simulink model "robocar_ss"  (R2024b)
settings: Solver=FixedStepAuto  StartTime=0  StopTime=5  FixedStep=0.001  RelTol=1e-3
libraries: slpidlib x4
settings Model: Creator=saucesaft  LastModifiedBy=saucesaft
settings HardwareCC: ProdBitPerLong=64  ProdHWDeviceType=Apple->ARM64

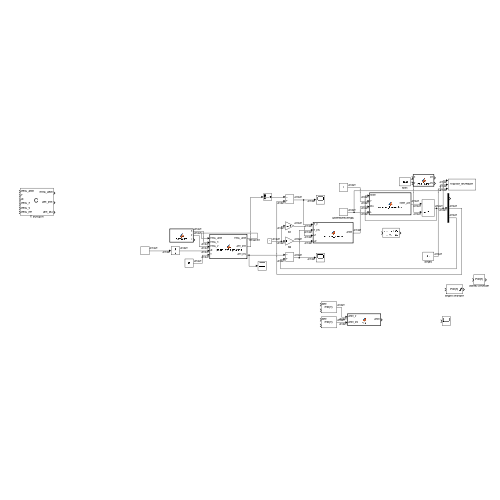
[thumbnail: Simulink's stored preview of the top-level diagram]
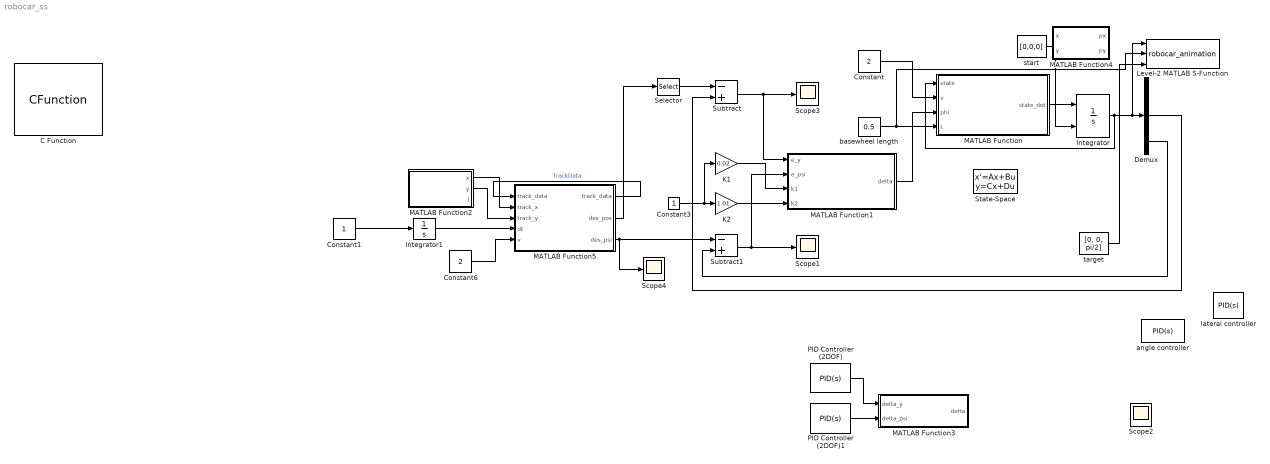
== system robocar_ss ==
  C Function : CFunction  OutputCode=|  InitializeConditionsCode=init = true;  CodegenOutputCode=|  CodegenInitializeConditionsCode=init = true;  SampleTime=0.01  CustomCodeSettingLocation=ModelConfigurationParameters
      OutputCode=|
      | #define MAX(x, y) (((x) > (y)) ? (x) : (y))
      | #define MIN(x, y) (((x) < (y)) ? (x) : (y))
      | 
      | if (init) {
      |     track_data.index = 1;
      |     track_data.t_marker = 0;
      | 
      |     track_data.A[0] = track_x[0];
      |     track_data.A[1] = track_y[0];
      | 
      |     track_data.B[0] = track_x[1];
      |     track_data.B[1] = track_y[1];
      |     
      |     init = false;
      | } 
      | 
      | double mag_vector[2];
      | mag_vector[0] = track_data.des_pos[0] - track_data.A[0];
      | mag_vector[1] = track_data.des_pos[1] - track_data.A[1];
      | 
      | double mag = sqrt( pow(mag_vector[0], 2) + pow(mag_vector[1], 2) );
      | 
      | if (mag >= track_data.base_norm) {
      |     track_data.index = MIN(track_data.index+1, track_len-1);
      |     
      |     mag_vector[0] = track_data.des_pos[0] - track_data.B[0];
      |     mag_vector[1] = track_data.des_pos[1] - track_data.B[1];
      |     track_data.t_marker = dt - (sqrt( pow(mag_vector[0], 2) + pow(mag_vector[1], 2) )/v);
      |     
      |     track_data.A[0] = track_x[track_data.index];
      |     track_data.A[1] = track_y[track_data.index];
      |     
      |     track_data.B[0] = track_x[track_data.index + 1];
      |     track_data.B[1] = track_y[track_data.index + 1];
      |     
      |     mag_vector[0] = track_data.B[0] - track_data.A[0];
      |     mag_vector[1] = track_data.B[1] - track_data.A[1];
      |     track_data.base_norm = sqrt( pow(mag_vector[0], 2) + pow(mag_vector[1], 2) );
      | }
      | 
      | mag_vector[0] = track_data.B[0] - track_data.A[0];
      | mag_vector[1] = track_data.B[1] - track_data.A[1];
      | mag = sqrt( pow(mag_vector[0], 2) + pow(mag_vector[1], 2) );
      | 
      | track_data.des_pos[0] = track_data.A[0] + v*(dt - track_data.t_marker) * (track_data.B[0]-track_data.A[0]) / mag;
      | track_data.des_pos[1] = track_data.A[1] + v*(dt - track_data.t_marker) * (track_data.B[1]-track_data.A[1]) / mag;
      | 
      | des_pos[0] = track_data.des_pos[0];
      | des_pos[1] = track_data.des_pos[1];
      | des_phi = atan2( track_data.B[1] - track_data.A[1], track_data.B[0] - track_data.A[0] );
      CodegenOutputCode=|
      | #define MAX(x, y) (((x) > (y)) ? (x) : (y))
      | #define MIN(x, y) (((x) < (y)) ? (x) : (y))
      | 
      | if (init) {
      |     track_data.index = 1;
      |     track_data.t_marker = 0;
      | 
      |     track_data.A[0] = track_x[0];
      |     track_data.A[1] = track_y[0];
      | 
      |     track_data.B[0] = track_x[1];
      |     track_data.B[1] = track_y[1];
      |     
      |     init = false;
      | } 
      | 
      | double mag_vector[2];
      | mag_vector[0] = track_data.des_pos[0] - track_data.A[0];
      | mag_vector[1] = track_data.des_pos[1] - track_data.A[1];
      | 
      | double mag = sqrt( pow(mag_vector[0], 2) + pow(mag_vector[1], 2) );
      | 
      | if (mag >= track_data.base_norm) {
      |     track_data.index = MIN(track_data.index+1, track_len-1);
      |     
      |     mag_vector[0] = track_data.des_pos[0] - track_data.B[0];
      |     mag_vector[1] = track_data.des_pos[1] - track_data.B[1];
      |     track_data.t_marker = dt - (sqrt( pow(mag_vector[0], 2) + pow(mag_vector[1], 2) )/v);
      |     
      |     track_data.A[0] = track_x[track_data.index];
      |     track_data.A[1] = track_y[track_data.index];
      |     
      |     track_data.B[0] = track_x[track_data.index + 1];
      |     track_data.B[1] = track_y[track_data.index + 1];
      |     
      |     mag_vector[0] = track_data.B[0] - track_data.A[0];
      |     mag_vector[1] = track_data.B[1] - track_data.A[1];
      |     track_data.base_norm = sqrt( pow(mag_vector[0], 2) + pow(mag_vector[1], 2) );
      | }
      | 
      | mag_vector[0] = track_data.B[0] - track_data.A[0];
      | mag_vector[1] = track_data.B[1] - track_data.A[1];
      | mag = sqrt( pow(mag_vector[0], 2) + pow(mag_vector[1], 2) );
      | 
      | track_data.des_pos[0] = track_data.A[0] + v*(dt - track_data.t_marker) * (track_data.B[0]-track_data.A[0]) / mag;
      | track_data.des_pos[1] = track_data.A[1] + v*(dt - track_data.t_marker) * (track_data.B[1]-track_data.A[1]) / mag;
      | 
      | des_pos[0] = track_data.des_pos[0];
      | des_pos[1] = track_data.des_pos[1];
      | des_phi = atan2( track_data.B[1] - track_data.A[1], track_data.B[0] - track_data.A[0] );
  Constant : Constant  Value=2
  Constant1 : Constant
  Constant3 : Constant
  Constant6 : Constant  Value=2
  Demux : Demux  Outputs=3
  Integrator : Integrator  InitialConditionSource=external  InitialCondition=[5,10,pi]
  Integrator1 : Integrator
  K1 : Gain  Gain=0.02
  K2 : Gain  Gain=1.01
  Level-2 MATLAB S-Function : M-S-Function  FunctionName=robocar_animation
  MATLAB Function : MATLAB Function  TreatAsAtomicUnit=on
  MATLAB Function1 : MATLAB Function  TreatAsAtomicUnit=on
  MATLAB Function2 : MATLAB Function  TreatAsAtomicUnit=on
  MATLAB Function3 : MATLAB Function  TreatAsAtomicUnit=on
  MATLAB Function4 : MATLAB Function  TreatAsAtomicUnit=on
  MATLAB Function5 : MATLAB Function  TreatAsAtomicUnit=on
  PID Controller (2DOF) : slpidlib/PID Controller (2DOF)  Controller=PID  Form=Parallel  TimeDomain=Continuous-time  UseExternalTs=off  SampleTime=-1  IntegratorMethod=Forward Euler  FilterMethod=Forward Euler  ControllerParametersSource=internal  P=1  I=1  UseKiTs=off  D=0  UseExternalDerivativeSource=off  N=100  UseFilter=on  b=1  c=1  TunerSelectOption=Transfer Function Based (PID Tuner App)  InitialConditionSource=internal  InitialConditionForIntegrator=0  InitialConditionForFilter=0  DifferentiatorICPrevScaledInput=0  ExternalReset=none  TrackingMode=off  Kt=1  LimitOutput=off  SatLimitsSource=internal  UpperSaturationLimit=inf  LowerSaturationLimit=-inf  LinearizeAsGain=on  AntiWindupMode=none  Kb=1  LimitIntegrator=off  UpperIntegratorSaturationLimit=inf  LowerIntegratorSaturationLimit=-inf  POutMin=[]  POutMax=[]  IOutMin=[]  IOutMax=[]  DOutMin=[]  DOutMax=[]  NOutMin=[]  NOutMax=[]  bOutMin=[]  bOutMax=[]  cOutMin=[]  cOutMax=[]  SumOutMin=[]  SumOutMax=[]  SaturationOutMin=[]  SaturationOutMax=[]  PParamMin=[]  PParamMax=[]  IParamMin=[]  IParamMax=[]  DParamMin=[]  DParamMax=[]  NParamMin=[]  NParamMax=[]  bParamMin=[]  bParamMax=[]  cParamMin=[]  cParamMax=[]  KbParamMin=[]  KbParamMax=[]  KtParamMin=[]  KtParamMax=[]  KbOutMin=[]  KbOutMax=[]  KtOutMin=[]  KtOutMax=[]  IntegratorOutMin=[]  IntegratorOutMax=[]  FilterOutMin=[]  FilterOutMax=[]  SumI1OutMin=[]  SumI1OutMax=[]  SumI2OutMin=[]  SumI2OutMax=[]  SumI3OutMin=[]  SumI3OutMax=[]  SumI4OutMin=[]  SumI4OutMax=[]  SumDOutMin=[]  SumDOutMax=[]  Sum1OutMin=[]  Sum1OutMax=[]  Sum2OutMin=[]  Sum2OutMax=[]  Sum3OutMin=[]  Sum3OutMax=[]  DifferentiatorOutMin=[]  DifferentiatorOutMax=[]  FilterDiffOutCoefMin=[]  FilterDiffOutCoefMax=[]  ReciprocalOutMin=[]  ReciprocalOutMax=[]  SumDenOutMin=[]  SumDenOutMax=[]  SumNumOutMin=[]  SumNumOutMax=[]  DivideOutMin=[]  DivideOutMax=[]  UdiffTsProdOutMin=[]  UdiffTsProdOutMax=[]  NTsProdOutMin=[]  NTsProdOutMax=[]  UintegralTsProdOutMin=[]  UintegralTsProdOutMax=[]  UngainTsProdOutMin=[]  UngainTsProdOutMax=[]  ClampingZeroOutDataTypeStr=Inherit: Inherit via back propagation  ClampingZeroOutMin=[]  ClampingZeroOutMax=[]  FilterDenConstantOutDataTypeStr=Inherit: Inherit via back propagation  FilterDenConstantOutMin=[]  FilterDenConstantOutMax=[]  PCopyOutDataTypeStr=Inherit: Inherit via back propagation  PCopyOutMin=[]  PCopyOutMax=[]  NCopyOutDataTypeStr=Inherit: Inherit via back propagation  NCopyOutMin=[]  NCopyOutMax=[]  IntegratorContinuousStateAttributes=''  IntegratorStateMustResolveToSignalObject=off  IntegratorRTWStateStorageClass=Auto  FilterContinuousStateAttributes=''  FilterStateMustResolveToSignalObject=off  FilterRTWStateStorageClass=Auto  ParallelPVariant=InternalParameters  IdealPVariant=Disabled  IVariant=InternalParameters  DVariant=InternalParameters  bVariant=InternalParameters  cVariant=InternalParameters  IntegratorVariant=Continuous  SatVariant=Disabled  AWVariant=Passthrough  PCopyVariant=Disabled  TRVariant=Disabled  FdbkBlocksVariant=Forward  IdealPFdbkVariant=Disabled  SatFdbkVariant=Disabled  DerivativeFilterVariant=ContFilter  NVariant=InternalParameters  NCopyVariant=Disabled  FilterICVariant=InternalICsFilter  IntegratorICVariant=InternalICs  ExternalResetVariant=Disabled  TRSumVariant=Passthrough  SumFdbkVariant=Disabled  SumVariant=Sum_PID  TsampFilterVariant=InternalTs  TsampNgainVariant=Passthrough  TsampIntegralVariant=Disabled_SignalSpec  ExternalSaturationOutDataTypeStr=Inherit: Same as second input  DerivativeSourceVariant=ErrorSignal  PreIntVariant=InternalPreInt
  PID Controller (2DOF)1 : slpidlib/PID Controller (2DOF)  Controller=PID  Form=Parallel  TimeDomain=Continuous-time  UseExternalTs=off  SampleTime=-1  IntegratorMethod=Forward Euler  FilterMethod=Forward Euler  ControllerParametersSource=internal  P=1  I=1  UseKiTs=off  D=0  UseExternalDerivativeSource=off  N=100  UseFilter=on  b=1  c=1  TunerSelectOption=Transfer Function Based (PID Tuner App)  InitialConditionSource=internal  InitialConditionForIntegrator=0  InitialConditionForFilter=0  DifferentiatorICPrevScaledInput=0  ExternalReset=none  TrackingMode=off  Kt=1  LimitOutput=off  SatLimitsSource=internal  UpperSaturationLimit=inf  LowerSaturationLimit=-inf  LinearizeAsGain=on  AntiWindupMode=none  Kb=1  LimitIntegrator=off  UpperIntegratorSaturationLimit=inf  LowerIntegratorSaturationLimit=-inf  POutMin=[]  POutMax=[]  IOutMin=[]  IOutMax=[]  DOutMin=[]  DOutMax=[]  NOutMin=[]  NOutMax=[]  bOutMin=[]  bOutMax=[]  cOutMin=[]  cOutMax=[]  SumOutMin=[]  SumOutMax=[]  SaturationOutMin=[]  SaturationOutMax=[]  PParamMin=[]  PParamMax=[]  IParamMin=[]  IParamMax=[]  DParamMin=[]  DParamMax=[]  NParamMin=[]  NParamMax=[]  bParamMin=[]  bParamMax=[]  cParamMin=[]  cParamMax=[]  KbParamMin=[]  KbParamMax=[]  KtParamMin=[]  KtParamMax=[]  KbOutMin=[]  KbOutMax=[]  KtOutMin=[]  KtOutMax=[]  IntegratorOutMin=[]  IntegratorOutMax=[]  FilterOutMin=[]  FilterOutMax=[]  SumI1OutMin=[]  SumI1OutMax=[]  SumI2OutMin=[]  SumI2OutMax=[]  SumI3OutMin=[]  SumI3OutMax=[]  SumI4OutMin=[]  SumI4OutMax=[]  SumDOutMin=[]  SumDOutMax=[]  Sum1OutMin=[]  Sum1OutMax=[]  Sum2OutMin=[]  Sum2OutMax=[]  Sum3OutMin=[]  Sum3OutMax=[]  DifferentiatorOutMin=[]  DifferentiatorOutMax=[]  FilterDiffOutCoefMin=[]  FilterDiffOutCoefMax=[]  ReciprocalOutMin=[]  ReciprocalOutMax=[]  SumDenOutMin=[]  SumDenOutMax=[]  SumNumOutMin=[]  SumNumOutMax=[]  DivideOutMin=[]  DivideOutMax=[]  UdiffTsProdOutMin=[]  UdiffTsProdOutMax=[]  NTsProdOutMin=[]  NTsProdOutMax=[]  UintegralTsProdOutMin=[]  UintegralTsProdOutMax=[]  UngainTsProdOutMin=[]  UngainTsProdOutMax=[]  ClampingZeroOutDataTypeStr=Inherit: Inherit via back propagation  ClampingZeroOutMin=[]  ClampingZeroOutMax=[]  FilterDenConstantOutDataTypeStr=Inherit: Inherit via back propagation  FilterDenConstantOutMin=[]  FilterDenConstantOutMax=[]  PCopyOutDataTypeStr=Inherit: Inherit via back propagation  PCopyOutMin=[]  PCopyOutMax=[]  NCopyOutDataTypeStr=Inherit: Inherit via back propagation  NCopyOutMin=[]  NCopyOutMax=[]  IntegratorContinuousStateAttributes=''  IntegratorStateMustResolveToSignalObject=off  IntegratorRTWStateStorageClass=Auto  FilterContinuousStateAttributes=''  FilterStateMustResolveToSignalObject=off  FilterRTWStateStorageClass=Auto  ParallelPVariant=InternalParameters  IdealPVariant=Disabled  IVariant=InternalParameters  DVariant=InternalParameters  bVariant=InternalParameters  cVariant=InternalParameters  IntegratorVariant=Continuous  SatVariant=Disabled  AWVariant=Passthrough  PCopyVariant=Disabled  TRVariant=Disabled  FdbkBlocksVariant=Forward  IdealPFdbkVariant=Disabled  SatFdbkVariant=Disabled  DerivativeFilterVariant=ContFilter  NVariant=InternalParameters  NCopyVariant=Disabled  FilterICVariant=InternalICsFilter  IntegratorICVariant=InternalICs  ExternalResetVariant=Disabled  TRSumVariant=Passthrough  SumFdbkVariant=Disabled  SumVariant=Sum_PID  TsampFilterVariant=InternalTs  TsampNgainVariant=Passthrough  TsampIntegralVariant=Disabled_SignalSpec  ExternalSaturationOutDataTypeStr=Inherit: Same as second input  DerivativeSourceVariant=ErrorSignal  PreIntVariant=InternalPreInt
  Scope{1..4} (4 alike) : Scope
  Selector : Selector  InputPortWidth=2  IndexOptions=Index vector (dialog)  Indices=2  OutputSizes=1
  State-Space : StateSpace  A=[0 10; 0 0]  B=[0; 10/1]  C=[1 0; 0 1]  D=[0; 0]  InitialCondition=0
  Subtract : Sum  Inputs=-+
  Subtract1 : Sum  Inputs=-+
  angle controller : slpidlib/PID Controller  Controller=PID  Form=Parallel  TimeDomain=Continuous-time  UseExternalTs=off  SampleTime=-1  IntegratorMethod=Forward Euler  FilterMethod=Forward Euler  ControllerParametersSource=internal  P=9.67739961508882  I=0.240279452636177  UseKiTs=off  D=100.4861253643554  UseExternalDerivativeSource=off  N=100  UseFilter=on  TunerSelectOption=Transfer Function Based (PID Tuner App)  InitialConditionSource=internal  InitialConditionForIntegrator=0  InitialConditionForFilter=0  DifferentiatorICPrevScaledInput=0  ExternalReset=none  TrackingMode=off  Kt=1  LimitOutput=on  SatLimitsSource=internal  UpperSaturationLimit=inf  LowerSaturationLimit=-inf  LinearizeAsGain=on  AntiWindupMode=back-calculation  Kb=1  LimitIntegrator=off  UpperIntegratorSaturationLimit=inf  LowerIntegratorSaturationLimit=-inf  POutMin=[]  POutMax=[]  IOutMin=[]  IOutMax=[]  DOutMin=[]  DOutMax=[]  NOutMin=[]  NOutMax=[]  SumOutMin=[]  SumOutMax=[]  SaturationOutMin=[]  SaturationOutMax=[]  PParamMin=[]  PParamMax=[]  IParamMin=[]  IParamMax=[]  DParamMin=[]  DParamMax=[]  NParamMin=[]  NParamMax=[]  KbParamMin=[]  KbParamMax=[]  KtParamMin=[]  KtParamMax=[]  KbOutMin=[]  KbOutMax=[]  KtOutMin=[]  KtOutMax=[]  IntegratorOutMin=[]  IntegratorOutMax=[]  FilterOutMin=[]  FilterOutMax=[]  SumI1OutMin=[]  SumI1OutMax=[]  SumI2OutMin=[]  SumI2OutMax=[]  SumI3OutMin=[]  SumI3OutMax=[]  SumI4OutMin=[]  SumI4OutMax=[]  SumDOutMin=[]  SumDOutMax=[]  DifferentiatorOutMin=[]  DifferentiatorOutMax=[]  FilterDiffOutCoefMin=[]  FilterDiffOutCoefMax=[]  ReciprocalOutMin=[]  ReciprocalOutMax=[]  SumDenOutMin=[]  SumDenOutMax=[]  SumNumOutMin=[]  SumNumOutMax=[]  DivideOutMin=[]  DivideOutMax=[]  UdiffTsProdOutMin=[]  UdiffTsProdOutMax=[]  NTsProdOutMin=[]  NTsProdOutMax=[]  UintegralTsProdOutMin=[]  UintegralTsProdOutMax=[]  UngainTsProdOutMin=[]  UngainTsProdOutMax=[]  ClampingZeroOutDataTypeStr=Inherit: Inherit via back propagation  ClampingZeroOutMin=[]  ClampingZeroOutMax=[]  FilterDenConstantOutDataTypeStr=Inherit: Inherit via back propagation  FilterDenConstantOutMin=[]  FilterDenConstantOutMax=[]  PCopyOutDataTypeStr=Inherit: Inherit via back propagation  PCopyOutMin=[]  PCopyOutMax=[]  NCopyOutDataTypeStr=Inherit: Inherit via back propagation  NCopyOutMin=[]  NCopyOutMax=[]  IntegratorContinuousStateAttributes=''  IntegratorStateMustResolveToSignalObject=off  IntegratorRTWStateStorageClass=Auto  FilterContinuousStateAttributes=''  FilterStateMustResolveToSignalObject=off  FilterRTWStateStorageClass=Auto  ParallelPVariant=InternalParameters  IdealPVariant=Disabled  IVariant=InternalParameters  DVariant=InternalParameters  IntegratorVariant=Continuous  SatVariant=Enabled  AWVariant=BackCalculation  PCopyVariant=Disabled  TRVariant=Disabled  FdbkBlocksVariant=Forward  IdealPFdbkVariant=Disabled  SatFdbkVariant=Disabled  DerivativeFilterVariant=ContFilter  NVariant=InternalParameters  NCopyVariant=Disabled  FilterICVariant=InternalICsFilter  IntegratorICVariant=InternalICs  ExternalResetVariant=Disabled  TRSumVariant=Passthrough  SumFdbkVariant=Disabled  SumVariant=Sum_PID  TsampFilterVariant=InternalTs  TsampNgainVariant=Passthrough  TsampIntegralVariant=Disabled_SignalSpec  ExternalSaturationOutDataTypeStr=Inherit: Same as second input  DerivativeSourceVariant=ErrorSignal  PreIntVariant=InternalPreInt
  basewheel length : Constant  Value=0.5
  lateral controller : slpidlib/PID Controller  Controller=PID  Form=Parallel  TimeDomain=Continuous-time  UseExternalTs=off  SampleTime=-1  IntegratorMethod=Forward Euler  FilterMethod=Forward Euler  ControllerParametersSource=internal  P=234  I=21  UseKiTs=off  D=4325  UseExternalDerivativeSource=off  N=100  UseFilter=on  TunerSelectOption=Transfer Function Based (PID Tuner App)  InitialConditionSource=internal  InitialConditionForIntegrator=0  InitialConditionForFilter=0  DifferentiatorICPrevScaledInput=0  ExternalReset=none  TrackingMode=off  Kt=1  LimitOutput=off  SatLimitsSource=internal  UpperSaturationLimit=inf  LowerSaturationLimit=-inf  LinearizeAsGain=on  AntiWindupMode=none  Kb=1  LimitIntegrator=off  UpperIntegratorSaturationLimit=inf  LowerIntegratorSaturationLimit=-inf  POutMin=[]  POutMax=[]  IOutMin=[]  IOutMax=[]  DOutMin=[]  DOutMax=[]  NOutMin=[]  NOutMax=[]  SumOutMin=[]  SumOutMax=[]  SaturationOutMin=[]  SaturationOutMax=[]  PParamMin=[]  PParamMax=[]  IParamMin=[]  IParamMax=[]  DParamMin=[]  DParamMax=[]  NParamMin=[]  NParamMax=[]  KbParamMin=[]  KbParamMax=[]  KtParamMin=[]  KtParamMax=[]  KbOutMin=[]  KbOutMax=[]  KtOutMin=[]  KtOutMax=[]  IntegratorOutMin=[]  IntegratorOutMax=[]  FilterOutMin=[]  FilterOutMax=[]  SumI1OutMin=[]  SumI1OutMax=[]  SumI2OutMin=[]  SumI2OutMax=[]  SumI3OutMin=[]  SumI3OutMax=[]  SumI4OutMin=[]  SumI4OutMax=[]  SumDOutMin=[]  SumDOutMax=[]  DifferentiatorOutMin=[]  DifferentiatorOutMax=[]  FilterDiffOutCoefMin=[]  FilterDiffOutCoefMax=[]  ReciprocalOutMin=[]  ReciprocalOutMax=[]  SumDenOutMin=[]  SumDenOutMax=[]  SumNumOutMin=[]  SumNumOutMax=[]  DivideOutMin=[]  DivideOutMax=[]  UdiffTsProdOutMin=[]  UdiffTsProdOutMax=[]  NTsProdOutMin=[]  NTsProdOutMax=[]  UintegralTsProdOutMin=[]  UintegralTsProdOutMax=[]  UngainTsProdOutMin=[]  UngainTsProdOutMax=[]  ClampingZeroOutDataTypeStr=Inherit: Inherit via back propagation  ClampingZeroOutMin=[]  ClampingZeroOutMax=[]  FilterDenConstantOutDataTypeStr=Inherit: Inherit via back propagation  FilterDenConstantOutMin=[]  FilterDenConstantOutMax=[]  PCopyOutDataTypeStr=Inherit: Inherit via back propagation  PCopyOutMin=[]  PCopyOutMax=[]  NCopyOutDataTypeStr=Inherit: Inherit via back propagation  NCopyOutMin=[]  NCopyOutMax=[]  IntegratorContinuousStateAttributes=''  IntegratorStateMustResolveToSignalObject=off  IntegratorRTWStateStorageClass=Auto  FilterContinuousStateAttributes=''  FilterStateMustResolveToSignalObject=off  FilterRTWStateStorageClass=Auto  ParallelPVariant=InternalParameters  IdealPVariant=Disabled  IVariant=InternalParameters  DVariant=InternalParameters  IntegratorVariant=Continuous  SatVariant=Disabled  AWVariant=Passthrough  PCopyVariant=Disabled  TRVariant=Disabled  FdbkBlocksVariant=Forward  IdealPFdbkVariant=Disabled  SatFdbkVariant=Disabled  DerivativeFilterVariant=ContFilter  NVariant=InternalParameters  NCopyVariant=Disabled  FilterICVariant=InternalICsFilter  IntegratorICVariant=InternalICs  ExternalResetVariant=Disabled  TRSumVariant=Passthrough  SumFdbkVariant=Disabled  SumVariant=Sum_PID  TsampFilterVariant=InternalTs  TsampNgainVariant=Passthrough  TsampIntegralVariant=Disabled_SignalSpec  ExternalSaturationOutDataTypeStr=Inherit: Same as second input  DerivativeSourceVariant=ErrorSignal  PreIntVariant=InternalPreInt
  start : Constant  Value=[0,0,0]
  target : Constant  Value=[0, 0, pi/2]
  wires:
  Demux/3 -> Subtract1/2
  target/1 -> Level-2 MATLAB S-Function/3
  MATLAB Function/1(state_dot) -> Integrator/1
  Subtract1/1 -> Scope1/1, MATLAB Function1/2(e_psi)
  basewheel length/1 -> MATLAB Function/4(L), Level-2 MATLAB S-Function/2
  Constant1/1 -> Integrator1/1
  K1/1 -> MATLAB Function1/3(k1)
  MATLAB Function2/1(x) -> MATLAB Function5/2(track_x)
  start/1 -> Integrator/2
  Demux/2 -> Subtract/2
  Subtract/1 -> Scope3/1, MATLAB Function1/1(e_y)
  Constant3/1 -> K1/1, K2/1
  Constant6/1 -> MATLAB Function5/5(v)
  Selector/1 -> Subtract/1
  MATLAB Function5/2(des_pos) -> Selector/1
  PID Controller (2DOF)/1 -> MATLAB Function3/1(delta_y)
  K2/1 -> MATLAB Function1/4(k2)
  MATLAB Function2/2(y) -> MATLAB Function5/3(track_y)
  Integrator/1 -> Demux/1, Level-2 MATLAB S-Function/1, MATLAB Function/1(state)
  PID Controller (2DOF)1/1 -> MATLAB Function3/2(delta_psi)
  Constant/1 -> MATLAB Function/2(v)
  Integrator1/1 -> MATLAB Function5/4(dt)
  MATLAB Function1/1(delta) -> MATLAB Function/3(phi)
  MATLAB Function5/3(des_psi) -> Scope4/1, Subtract1/1
  MATLAB Function5/1(track_data) -> MATLAB Function5/1("track_data ")  "TrackData"

== matlab function robocar_ss/MATLAB Function1 ==
  data: e_y input; delta output; e_psi input; k1 input; k2 input
function delta = calculate_steering(e_y, e_psi, k1, k2)
    delta = -k1 * e_y - k2 * e_psi;
    delta = max(min(delta, 0.5), -0.5);
end

== matlab function robocar_ss/MATLAB Function ==
  data: state input; state_dot output; v input; phi input; L input
function state_dot = robocar_kinematics(state, v, phi, L)
    % state = [x; y; theta]
    % L = wheelbase length

    theta = state(3);

    x_dot = v * cos(theta);
    y_dot = v * sin(theta);
    theta_dot = (v/L) * tan(phi);

    state_dot = [x_dot, y_dot, theta_dot];
end

== matlab function robocar_ss/MATLAB Function2 ==
  data: x output; y output; l output
function [x, y, l] = setpoints()
    % xd1 = [0.0 2.0 10.0 14.0 15.0];    % Coordinates of bottom half
    % yd1 = [0 0 3.0 10.0 15.0];         % Coordinates of bottom half
    % xd22 = [0 2.0 10.0 15.0];          % Coordinates of upper half
    % yd22 = [30.0 30.0 27.0 20.0];      % Coordinates of upper half
    % 
    % xd2 = fliplr(xd22);
    % yd2 = fliplr(yd22);
    % 
    % x = [xd1, xd2];
    % y = [yd1, yd2];
    % l = length(x);

    x = [0.0 2.0 0.0];
    y = [0.0 2.0 4.0];
    l = length(x);
end

== matlab function robocar_ss/MATLAB Function3 ==
  data: delta_y input; delta output; delta_psi input
function delta = fcn(delta_y, delta_psi)
    delta = delta_y + delta_psi;
    delta = max(min(delta, 0.5), -0.5);

== matlab function robocar_ss/MATLAB Function4 ==
  data: x input; px output; y input; py output
function [px, py] = pad_track(x, y)
    px = zeros(1, 256);
    px(1, 1:numel(x)) = x;
    
    py = zeros(1, 256);
    py(1, 1:numel(y)) = y;
end

== matlab function robocar_ss/MATLAB Function5 ==
  data: track_data input; track_data output; track_x input; track_y input; dt input; v input; des_pos output; des_psi output
function [track_data, des_pos, des_psi] = update_track_position(track_data, track_x, track_y, dt, v)

    % Update desired position along the track
    if norm(track_data.des_pos - track_data.A) >= track_data.base_norm
        track_data.index = min(track_data.index + 1, length(track_x) - 1);
        track_data.t_marker = dt - (norm(track_data.des_pos - track_data.B)/v);
        track_data.A = [track_x(track_data.index); track_y(track_data.index)];
        track_data.B = [track_x(track_data.index + 1); track_y(track_data.index + 1)];
        track_data.base_norm = norm(track_data.B - track_data.A);
    end
    
    % if v == 0
    %     % If stopped, stay at current position
    %     track_data.des_pos = track_data.des_pos;
    % else
        % Normal update of desired position
        track_data.des_pos = track_data.A + v*(dt - track_data.t_marker)* ...
                            (track_data.B - track_data.A)./norm(track_data.B - track_data.A);
    % end
    
    des_pos = track_data.des_pos;
    des_psi = atan2((track_data.B(2) - track_data.A(2)), (track_data.B(1) - track_data.A(1)));
end
